simulink model "six_plus_six_AcmsteeringV09_main_2lflm"  (R2014a)
settings: Solver=FixedStepDiscrete  StartTime=0.0  StopTime=10.0  FixedStep=0.0005  RelTol=1e-3
InitFcn:
  | Veh_Par_wxt
undefined symbols (not defined in the file or in its folder): acc_spdctl, ag_thr, B, bra_em, bra_pre_gz2, bra_pre_gz34, bra_pre_yd, brakepre_dem_data, brakeTrq_dem_data, bratrq_max, ecucoder_acal, eff_tran, ESP_switch, G, guzhang_lf, guzhang_lm, guzhang_lr, guzhang_rf, guzhang_rm, guzhang_rr, kd1, kd2, ki1, ki2, kp1, kp2, L, myFIS, premax, Radius, RC_switch, s_opt_yi, s_opt_zhuan, s_opt_zhuan_add, s_opt_zhuan_table, spd_map_mot, spd_spdctl, speed_thr_park, TCS_switch, tras_ratio, trq_map_mot, trqmax_yd, trqmax_zx, trqmaxneg, v_gain, v_table, v_thr_park, zhidong_bianmazhi, zhidong_down, zhidong_up, zhidong_youmen, zhuanxiang_bianmazhi, zhuanxiang_down, zhuanxiang_up, zhuanxiang_youmen
libraries: simulink x980, ec5744lib x59, fuzblock x2
(part 21 of 25)

== system six_plus_six_AcmsteeringV09_main_2lflm/MainControl/mode_control/backward/backward/Drive/目标直驶力矩确定模块 ==
  acc_dem : Inport
  TrqLimU_dig_lf : Inport  Port=2
  TrqLimU_dig_lm : Inport  Port=3
  TrqLimU_dig_lr : Inport  Port=4
  TrqLimU_dig_rf : Inport  Port=5
  TrqLimU_dig_rm : Inport  Port=6
  TrqLimU_dig_rr : Inport  Port=7
  speed_act_lf : Inport  Port=8
  speed_act_lm : Inport  Port=9
  speed_act_lr : Inport  Port=10
  speed_act_rf : Inport  Port=11
  speed_act_rm : Inport  Port=12
  speed_act_rr : Inport  Port=13
  Add : Sum  Inputs=++++++
  Constant : Constant  Value=3.6  OutDataTypeStr=single  SampleTime=-1
  Constant1 : Constant  Value=Radius  OutDataTypeStr=single  SampleTime=-1
  Constant2 : Constant  Value=30/pi  OutDataTypeStr=single  SampleTime=-1
  Divide : Product  Inputs=*//*
  Gain : Gain  Gain=1/100
  Gain1 : Gain  Gain=tras_ratio
  Ground : Ground
  MinMax{,1..5} (6 alike) : MinMax  Inputs=2
  Product : Product
  Terminator : Terminator
  mot_map{,1..5} (6 alike) : Lookup_n-D  NumberOfTableDimensions=1  BreakpointsForDimension1=spd_map_mot  Table=trq_map_mot  InternalRulePriority=Speed  RndMeth=Simplest  InputSameDT=on
  Trq_line_dem : Outport
  wires:
  Constant1/1 -> Divide/3
  Constant/1 -> Divide/2
  Constant2/1 -> Divide/4
  Divide/1 -> Gain1/1
  TrqLimU_dig_lf/1 -> MinMax/2
  mot_map/1 -> MinMax/1
  TrqLimU_dig_lm/1 -> MinMax1/2
  TrqLimU_dig_rm/1 -> MinMax2/2
  TrqLimU_dig_rr/1 -> MinMax3/2
  Add/1 -> Product/2
  acc_dem/1 -> Gain/1
  Gain/1 -> Product/1
  Ground/1 -> Divide/1
  Gain1/1 -> Terminator/1
  speed_act_lf/1 -> mot_map/1
  speed_act_lm/1 -> mot_map1/1
  speed_act_rm/1 -> mot_map2/1
  speed_act_rr/1 -> mot_map3/1
  mot_map1/1 -> MinMax1/1
  mot_map2/1 -> MinMax2/1
  mot_map3/1 -> MinMax3/1
  Product/1 -> Trq_line_dem/1
  TrqLimU_dig_lr/1 -> MinMax4/2
  mot_map4/1 -> MinMax4/1
  TrqLimU_dig_rf/1 -> MinMax5/2
  speed_act_lr/1 -> mot_map4/1
  speed_act_rf/1 -> mot_map5/1
  mot_map5/1 -> MinMax5/1
  MinMax1/1 -> Add/2
  MinMax/1 -> Add/1
  MinMax4/1 -> Add/3
  MinMax5/1 -> Add/4
  MinMax2/1 -> Add/5
  MinMax3/1 -> Add/6

== system six_plus_six_AcmsteeringV09_main_2lflm/MainControl/mode_control/backward/backward/Drive/目标转向力矩确定模块 ==
  note: 左转为正，右转为负
  TrqLimU_dig_lf : Inport
  TrqLimU_dig_lm : Inport  Port=2
  TrqLimU_dig_lr : Inport  Port=3
  TrqLimU_dig_rf : Inport  Port=4
  TrqLimU_dig_rm : Inport  Port=5
  TrqLimU_dig_rr : Inport  Port=6
  steer_dem : Inport  Port=7
  umax : Inport  Port=8
  f : Inport  Port=9
  speed_act_lf : Inport  Port=10
  speed_act_lm : Inport  Port=11
  speed_act_lr : Inport  Port=12
  speed_act_rf : Inport  Port=13
  speed_act_rm : Inport  Port=14
  speed_act_rr : Inport  Port=15
  Add : Sum  Inputs=+++
  Add1 : Sum  Inputs=+++
  Add2 : Sum  Inputs=++++++
  Constant : Constant  Value=3.6  OutDataTypeStr=single  SampleTime=-1
  Constant1 : Constant  Value=Radius  OutDataTypeStr=single  SampleTime=-1
  Constant2 : Constant  Value=30/pi  OutDataTypeStr=single  SampleTime=-1
  Constant3 : Constant  Value=G  OutDataTypeStr=single  SampleTime=-1
  Constant4 : Constant  Value=L  OutDataTypeStr=single  SampleTime=-1
  Constant5 : Constant  Value=B  OutDataTypeStr=single  SampleTime=-1
  Constant6 : Constant  Value=eff_tran  OutDataTypeStr=single  SampleTime=-1
  Constant7 : Constant  Value=Radius  OutDataTypeStr=single  SampleTime=-1
  Constant8 : Constant  Value=ag_thr  OutDataTypeStr=single  SampleTime=-1
  Constant9 : Constant  Value=Radius  OutDataTypeStr=single  SampleTime=-1
  Divide : Product  Inputs=*//*
  Gain : Gain  Gain=1/100
  Gain1 : Gain  Gain=tras_ratio
  Gain10 : Gain  Gain=3.6
  Gain2 : Gain  Gain=tras_ratio  OutDataTypeStr=single
  Gain3 : Gain  Gain=1/tras_ratio
  Gain4 : Gain  Gain=tras_ratio  OutDataTypeStr=single
  Gain6 : Gain  Gain=1/6
  Gain7 : Gain  Gain=1/tras_ratio
  Gain8 : Gain  Gain=pi/30
  Gain9 : Gain  Gain=Radius
  Ground : Ground
  MATLAB Function : MATLAB Function  TreatAsAtomicUnit=on
  MATLAB Function1 : MATLAB Function  TreatAsAtomicUnit=on
  MATLAB Function2 : MATLAB Function  TreatAsAtomicUnit=on
  MinMax{,1..3,5..6} (6 alike) : MinMax  Inputs=2
  MinMax4 : MinMax  Function=max  Inputs=2
  Product : Product
  Terminator : Terminator
  mot_map{,1..5} (6 alike) : Lookup_n-D  NumberOfTableDimensions=1  BreakpointsForDimension1=spd_map_mot  Table=trq_map_mot  InternalRulePriority=Speed  RndMeth=Simplest  InputSameDT=on
  delta_Tsteer_dem : Outport
  wires:
  Gain/1 -> Product/1
  Product/1 -> Gain3/1
  [steer_dem] -> Gain/1
  MinMax3/1 -> Add1/2
  MinMax/1 -> Add/1
  MinMax2/1 -> Add1/1
  MinMax1/1 -> Add/2
  TrqLimU_dig_rm/1 -> MinMax3/2
  TrqLimU_dig_rf/1 -> MinMax2/2
  TrqLimU_dig_lm/1 -> MinMax1/2
  mot_map/1 -> MinMax/1
  TrqLimU_dig_lf/1 -> MinMax/2
  Divide/1 -> Gain1/1
  Constant2/1 -> Divide/4
  Constant/1 -> Divide/2
  Constant1/1 -> Divide/3
  steer_dem/1 -> [steer_dem], MATLAB Function/1(steer_dem)
  Constant3/1 -> [G], MATLAB Function/2(G)
  Constant4/1 -> [L], MATLAB Function/3(L)
  Constant5/1 -> [B], MATLAB Function/5(B)
  umax/1 -> [umax], MATLAB Function/4(umax)
  Add/1 -> Gain2/1
  Add1/1 -> Gain4/1
  Constant6/1 -> MATLAB Function/8(eff_tran)
  Constant7/1 -> MATLAB Function/9(Radius)
  f/1 -> MATLAB Function/10(f)
  MATLAB Function/1(Rturn_min) -> MinMax4/1
  [v_act] -> MATLAB Function1/1(v_act)
  Constant8/1 -> MATLAB Function1/2(ag_thr)
  MATLAB Function1/1(Rturn_min_ag) -> MinMax4/2
  [umax] -> MATLAB Function2/1(umax)
  [G] -> MATLAB Function2/2(G)
  [L] -> MATLAB Function2/3(L)
  [B] -> MATLAB Function2/4(B)
  Constant9/1 -> MATLAB Function2/5(Radius)
  MinMax4/1 -> MATLAB Function2/6(Rturn_min_xy)
  MATLAB Function2/1(delta_Tsteer_max) -> Product/2
  Ground/1 -> Divide/1
  Gain2/1 -> MATLAB Function/6(Tpeak_L)
  Gain4/1 -> MATLAB Function/7(Tpeak_R)
  speed_act_lm/1 -> Add2/2, mot_map2/1
  speed_act_rf/1 -> Add2/4, mot_map3/1
  speed_act_rm/1 -> Add2/5, mot_map4/1
  Gain1/1 -> Terminator/1
  speed_act_lf/1 -> Add2/1, mot_map/1
  mot_map2/1 -> MinMax1/1
  mot_map3/1 -> MinMax2/1
  mot_map4/1 -> MinMax3/1
  Gain3/1 -> delta_Tsteer_dem/1
  MinMax5/1 -> Add/3
  TrqLimU_dig_lr/1 -> MinMax5/2
  speed_act_lr/1 -> Add2/3, mot_map1/1
  mot_map1/1 -> MinMax5/1
  MinMax6/1 -> Add1/3
  TrqLimU_dig_rr/1 -> MinMax6/2
  speed_act_rr/1 -> Add2/6, mot_map5/1
  mot_map5/1 -> MinMax6/1
  Add2/1 -> Gain6/1
  Gain6/1 -> Gain7/1
  Gain7/1 -> Gain8/1
  Gain8/1 -> Gain9/1
  Gain9/1 -> Gain10/1
  Gain10/1 -> [v_act]

== system six_plus_six_AcmsteeringV09_main_2lflm/MainControl/mode_control/backward/backward/Drive/路面状况识别模块 ==
  In1 : Inport
  miu : Inport  Port=2
  slip_ratio : Inport  Port=3
  Signals : Inport  Port=4
  1-D Lookup Table : Lookup_n-D  NumberOfTableDimensions=1  BreakpointsForDimension1=v_table  Table=s_opt_zhuan_table  InternalRulePriority=Speed  RndMeth=Simplest  InputSameDT=on
  Abs{11..14,19..20} (6 alike) : Abs  OutDataTypeStr=single
  Bus Selector8 : BusSelector  OutputSignals=MOTOR.MOTOR1.MCU0.MCU0_SpeedFdk,MOTOR.MOTOR3.MCU0_2.MCU0_2SpeedFdk,MOTOR.MOTOR5.MCU0_4.MCU0_4SpeedFdk,MOTOR.MOTOR2.MCU0_1.MCU0_1SpeedFdk,MOTOR.MOTOR4.MCU0_3.MCU0_3SpeedFdk,MOTOR.MOTOR6.MCU0_5.MCU0_5SpeedFdk
  Constant : Constant  Value=0.9  OutDataTypeStr=single  SampleTime=-1
  Constant1 : Constant  Value=0.05  OutDataTypeStr=single  SampleTime=-1
  Constant2 : Constant  Value=s_opt_zhuan  OutDataTypeStr=single  SampleTime=-1
  Constant3 : Constant  Value=s_opt_yi  OutDataTypeStr=single  SampleTime=-1
  Gain1 : Gain  Gain=1/tras_ratio
  Gain2 : Gain  Gain=pi/30
  Gain3 : Gain  Gain=Radius
  Gain4 : Gain  Gain=3.6
  Gain5 : Gain  Gain=v_gain
  MinMax : MinMax  Inputs=6
  Terminator{,1..3} (4 alike) : Terminator
  路面识别模块 : Subsystem  Commented=on
  umax : Outport
  f : Outport  Port=2
  s_opt_zhuan : Outport  Port=3
  s_opt_yi : Outport  Port=4
  wires:
  Constant/1 -> umax/1
  Constant1/1 -> f/1
  Constant2/1 -> Terminator3/1
  Constant3/1 -> s_opt_yi/1
  In1/1 -> Terminator/1
  miu/1 -> 路面识别模块/1(miu)
  slip_ratio/1 -> 路面识别模块/2(slip_ratio)
  路面识别模块/1(best_slip_ratio) -> Terminator1/1
  路面识别模块/2(max_miu) -> Terminator2/1
  Signals/1 -> Bus Selector8/1
  Abs12/1 -> MinMax/2
  Abs11/1 -> MinMax/1
  Abs13/1 -> MinMax/3
  Abs14/1 -> MinMax/4
  Abs19/1 -> MinMax/5
  Abs20/1 -> MinMax/6
  Bus Selector8/2 -> Abs12/1  "<MCU0_2SpeedFdk>"
  Bus Selector8/1 -> Abs11/1  "<MCU0_SpeedFdk>"
  Bus Selector8/3 -> Abs13/1  "<MCU0_4SpeedFdk>"
  Bus Selector8/4 -> Abs14/1  "<MCU0_1SpeedFdk>"
  Bus Selector8/5 -> Abs19/1  "<MCU0_3SpeedFdk>"
  Bus Selector8/6 -> Abs20/1  "<MCU0_5SpeedFdk>"
  MinMax/1 -> Gain1/1
  Gain1/1 -> Gain2/1
  Gain2/1 -> Gain3/1
  Gain3/1 -> Gain4/1
  Gain4/1 -> Gain5/1
  Gain5/1 -> 1-D Lookup Table/1
  1-D Lookup Table/1 -> s_opt_zhuan/1

== system six_plus_six_AcmsteeringV09_main_2lflm/MainControl/mode_control/backward/backward/Drive/车辆稳定性控制 ==
  note: 加速度向左为正
  acc_y : Inport
  Action Port : ActionPort  ActionType=case
  Abs : Abs
  Add10 : Sum  Inputs=+-+
  Add2 : Sum  Inputs=+++
  Constant : Constant  Value=ag_thr  OutDataTypeStr=single  SampleTime=-1
  Constant1 : Constant  OutDataTypeStr=int8  SampleTime=-1
  Constant2 : Constant  Value=-1  OutDataTypeStr=int8  SampleTime=-1
  Constant3 : Constant  Value=ESP_switch  OutDataTypeStr=single  SampleTime=-1
  Constant4 : Constant  Value=0  OutDataTypeStr=single  SampleTime=-1
  Gain20 : Gain  Gain=2
  Gain3 : Gain  Gain=1/tras_ratio
  Gain5 : Gain  Gain=kp1  OutDataTypeStr=single
  Gain6 : Gain  Gain=ki1  OutDataTypeStr=single
  Gain7 : Gain  Gain=kd1  OutDataTypeStr=single
  Memory{3..5,13} (4 alike) : Memory  InheritSampleTime=on
  Product : Product  OutDataTypeStr=single
  Subtract1 : Sum  Inputs=+-
  Subtract5 : Sum
  Sum : Sum  Inputs=|+-
  Switch : Switch
  Switch1 : Switch  Criteria=u2 > Threshold  Threshold=0.5
  delta_Twending_dem : Outport
  wires:
  Constant/1 -> Sum/1
  acc_y/1 -> Switch/2, Abs/1
  Abs/1 -> Sum/2
  Constant1/1 -> Switch/1
  Constant2/1 -> Switch/3
  Switch/1 -> Product/2
  Product/1 -> Gain3/1
  Constant3/1 -> Switch1/2
  Switch1/1 -> delta_Twending_dem/1
  Constant4/1 -> Switch1/3
  Sum/1 -> Memory4/1, Add10/1, Gain6/1, Memory3/1, Subtract1/1
  Gain5/1 -> Add2/1
  Gain6/1 -> Add2/2
  Memory3/1 -> Subtract1/2
  Add10/1 -> Gain7/1
  Gain20/1 -> Add10/2
  Memory5/1 -> Add10/3
  Gain7/1 -> Add2/3
  Subtract1/1 -> Gain5/1
  Memory4/1 -> Memory5/1, Gain20/1
  Add2/1 -> Subtract5/1
  Subtract5/1 -> Product/1, Memory13/1
  Memory13/1 -> Subtract5/2
  Gain3/1 -> Switch1/1

== system six_plus_six_AcmsteeringV09_main_2lflm/MainControl/mode_control/backward/backward/Drive/车辆稳定性控制1 ==
  Action Port : ActionPort  ActionType=case
  Constant4 : Constant  Value=0  OutDataTypeStr=single  SampleTime=-1
  1 : Outport
  wires:
  Constant4/1 -> 1/1

== system six_plus_six_AcmsteeringV09_main_2lflm/MainControl/mode_control/backward/backward/Drive/驱动防滑控制TCS ==
  trq_dem_lf : Inport
  trq_dem_lm : Inport  Port=2
  trq_dem_lr : Inport  Port=3
  trq_dem_rf : Inport  Port=4
  trq_dem_rm : Inport  Port=5
  trq_dem_rr : Inport  Port=6
  bra_pre_l : Inport  Port=7
  bra_pre_r : Inport  Port=8
  speed_act_lf : Inport  Port=9
  speed_act_lm : Inport  Port=10
  speed_act_lr : Inport  Port=11
  speed_act_rf : Inport  Port=12
  speed_act_rm : Inport  Port=13
  speed_act_rr : Inport  Port=14
  v_act : Inport  Port=15
  brake_dem : Inport  Port=16
  s_opt_zhuan : Inport  Port=17
  Signals : Inport  Port=18
  直行TCS : Subsystem  TreatAsAtomicUnit=on
  backward_dem : Outport
  wires:
  直行TCS/1(backward_dem) -> backward_dem/1
  trq_dem_lf/1 -> 直行TCS/1(trq_dem_lf)
  trq_dem_lm/1 -> 直行TCS/2(trq_dem_lm)
  trq_dem_lr/1 -> 直行TCS/3(trq_dem_lr)
  trq_dem_rf/1 -> 直行TCS/4(trq_dem_rf)
  trq_dem_rm/1 -> 直行TCS/5(trq_dem_rm)
  trq_dem_rr/1 -> 直行TCS/6(trq_dem_rr)
  bra_pre_l/1 -> 直行TCS/7(bra_pre_l)
  bra_pre_r/1 -> 直行TCS/8(bra_pre_r)
  brake_dem/1 -> 直行TCS/16(brake_dem)
  Signals/1 -> 直行TCS/18(Signals)
  speed_act_rr/1 -> 直行TCS/14(speed_act_rr)
  speed_act_rm/1 -> 直行TCS/13(speed_act_rm)
  v_act/1 -> 直行TCS/15(v_act)
  speed_act_rf/1 -> 直行TCS/12(speed_act_rf)
  speed_act_lr/1 -> 直行TCS/11(speed_act_lr)
  speed_act_lm/1 -> 直行TCS/10(speed_act_lm)
  speed_act_lf/1 -> 直行TCS/9(speed_act_lf)
  s_opt_zhuan/1 -> 直行TCS/17(s_opt_zhuan)

== system six_plus_six_AcmsteeringV09_main_2lflm/MainControl/mode_control/forward/forward/Brake/Subsystem ==
  MCU2 : Inport
  Bus Selector : BusSelector  OutputSignals=MCU2_MotorStallingFault,MCU2_UdcDetectionFault,MCU2_TempSensorFault,MCU2_ActiveDischargingFault,MCU2_ldcSensorFault,MCU2_luSensorFault,MCU2_lvSensorFault,MCU2_FaultLevel,MCU2_Controllerload,MCU2_CanCommunicationFault,MCU2_MemoryFault,MCU2_DownratingFault,MCU2_IGBTFault,MCU2_MotorOverTemp,MCU2_ControllerOverTemp,MCU2_MotorOverSpeed,MCU2_RotaryInverterFault,MCU2_UnderVoltage,MCU2_OverVoltage,MCU2_MotorOverLoad
  Compare To Constant{,1..19} (20 alike) : simulink/Logic and Bit Operations/Compare To Constant  relop===  const=1  OutDataTypeStr=boolean
  Logical Operator : Logic  Operator=OR  Inputs=20  AllPortsSameDT=off  OutDataTypeStr=boolean
  guzhang_lf : Outport
  wires:
  MCU2/1 -> Bus Selector/1
  Bus Selector/1 -> Compare To Constant/1  "<MCU2_MotorStallingFault>"
  Bus Selector/2 -> Compare To Constant1/1  "<MCU2_UdcDetectionFault>"
  Bus Selector/3 -> Compare To Constant2/1  "<MCU2_TempSensorFault>"
  Bus Selector/4 -> Compare To Constant3/1  "<MCU2_ActiveDischargingFault>"
  Bus Selector/5 -> Compare To Constant4/1  "<MCU2_ldcSensorFault>"
  Bus Selector/6 -> Compare To Constant5/1  "<MCU2_luSensorFault>"
  Bus Selector/7 -> Compare To Constant6/1  "<MCU2_lvSensorFault>"
  Bus Selector/8 -> Compare To Constant7/1  "<MCU2_FaultLevel>"
  Bus Selector/13 -> Compare To Constant12/1  "<MCU2_IGBTFault>"
  Bus Selector/14 -> Compare To Constant13/1  "<MCU2_MotorOverTemp>"
  Bus Selector/10 -> Compare To Constant9/1  "<MCU2_CanCommunicationFault>"
  Bus Selector/16 -> Compare To Constant15/1  "<MCU2_MotorOverSpeed>"
  Bus Selector/11 -> Compare To Constant10/1  "<MCU2_MemoryFault>"
  Bus Selector/15 -> Compare To Constant14/1  "<MCU2_ControllerOverTemp>"
  Bus Selector/12 -> Compare To Constant11/1  "<MCU2_DownratingFault>"
  Bus Selector/9 -> Compare To Constant8/1  "<MCU2_Controllerload>"
  Bus Selector/18 -> Compare To Constant17/1  "<MCU2_UnderVoltage>"
  Bus Selector/20 -> Compare To Constant19/1  "<MCU2_MotorOverLoad>"
  Bus Selector/19 -> Compare To Constant18/1  "<MCU2_OverVoltage>"
  Bus Selector/17 -> Compare To Constant16/1  "<MCU2_RotaryInverterFault>"
  Compare To Constant9/1 -> Logical Operator/10
  Compare To Constant12/1 -> Logical Operator/13
  Compare To Constant11/1 -> Logical Operator/12
  Compare To Constant15/1 -> Logical Operator/16
  Compare To Constant8/1 -> Logical Operator/9
  Compare To Constant10/1 -> Logical Operator/11
  Compare To Constant13/1 -> Logical Operator/14
  Compare To Constant14/1 -> Logical Operator/15
  Compare To Constant1/1 -> Logical Operator/2
  Compare To Constant17/1 -> Logical Operator/18
  Compare To Constant16/1 -> Logical Operator/17
  Compare To Constant18/1 -> Logical Operator/19
  Compare To Constant19/1 -> Logical Operator/20
  Compare To Constant3/1 -> Logical Operator/4
  Compare To Constant2/1 -> Logical Operator/3
  Compare To Constant6/1 -> Logical Operator/7
  Compare To Constant4/1 -> Logical Operator/5
  Compare To Constant5/1 -> Logical Operator/6
  Compare To Constant7/1 -> Logical Operator/8
  Compare To Constant/1 -> Logical Operator/1
  Logical Operator/1 -> guzhang_lf/1

== system six_plus_six_AcmsteeringV09_main_2lflm/MainControl/mode_control/forward/forward/Brake/Subsystem1 ==
  speed_act_lf : Inport
  speed_act_lm : Inport  Port=2
  speed_act_lr : Inport  Port=3
  speed_act_rf : Inport  Port=4
  speed_act_rm : Inport  Port=5
  speed_act_rr : Inport  Port=6
  mot_map{,1..5} (6 alike) : Lookup_n-D  NumberOfTableDimensions=1  BreakpointsForDimension1=spd_map_mot  Table=trq_map_mot  InternalRulePriority=Speed  RndMeth=Simplest  InputSameDT=on
  trqlim_map_lf : Outport
  trqlim_map_lm : Outport  Port=2
  trqlim_map_lr : Outport  Port=3
  trqlim_map_rf : Outport  Port=4
  trqlim_map_rm : Outport  Port=5
  trqlim_map_rr : Outport  Port=6
  wires:
  speed_act_lf/1 -> mot_map/1
  speed_act_lr/1 -> mot_map1/1
  speed_act_rf/1 -> mot_map2/1
  speed_act_rr/1 -> mot_map3/1
  mot_map/1 -> trqlim_map_lf/1
  mot_map1/1 -> trqlim_map_lr/1
  mot_map2/1 -> trqlim_map_rf/1
  mot_map3/1 -> trqlim_map_rr/1
  speed_act_lm/1 -> mot_map4/1
  mot_map4/1 -> trqlim_map_lm/1
  speed_act_rm/1 -> mot_map5/1
  mot_map5/1 -> trqlim_map_rm/1

== system six_plus_six_AcmsteeringV09_main_2lflm/MainControl/mode_control/forward/forward/Brake/Subsystem2 ==
  MCU2_2 : Inport
  Bus Selector : BusSelector  OutputSignals=MCU2_2MotorStallingFault,MCU2_2UdcDetectionFault,MCU2_2TempSensorFault,MCU2_2ActiveDischargingFault,MCU2_2ldcSensorFault,MCU2_2luSensorFault,MCU2_2lvSensorFault,MCU2_2FaultLevel,MCU2_2Controllerload,MCU2_2CanCommunicationFault,MCU2_2MemoryFault,MCU2_2DownratingFault,MCU2_2IGBTFault,MCU2_2MotorOverTemp,MCU2_2ControllerOverTemp,MCU2_2MotorOverSpeed,MCU2_2RotaryInverterFault,MCU2_2UnderVoltage,MCU2_OverVoltage,MCU2_2MotorOverLoad
  Compare To Constant{,1..19} (20 alike) : simulink/Logic and Bit Operations/Compare To Constant  relop===  const=1  OutDataTypeStr=boolean
  Logical Operator : Logic  Operator=OR  Inputs=20  AllPortsSameDT=off  OutDataTypeStr=boolean
  guzhang_lm : Outport
  wires:
  Logical Operator/1 -> guzhang_lm/1
  Compare To Constant/1 -> Logical Operator/1
  Compare To Constant7/1 -> Logical Operator/8
  Compare To Constant5/1 -> Logical Operator/6
  Compare To Constant4/1 -> Logical Operator/5
  Compare To Constant6/1 -> Logical Operator/7
  Compare To Constant2/1 -> Logical Operator/3
  Compare To Constant3/1 -> Logical Operator/4
  Compare To Constant19/1 -> Logical Operator/20
  Compare To Constant18/1 -> Logical Operator/19
  Compare To Constant16/1 -> Logical Operator/17
  Compare To Constant17/1 -> Logical Operator/18
  Compare To Constant1/1 -> Logical Operator/2
  Compare To Constant14/1 -> Logical Operator/15
  Compare To Constant13/1 -> Logical Operator/14
  Compare To Constant10/1 -> Logical Operator/11
  Compare To Constant8/1 -> Logical Operator/9
  Compare To Constant15/1 -> Logical Operator/16
  Compare To Constant11/1 -> Logical Operator/12
  Compare To Constant12/1 -> Logical Operator/13
  Compare To Constant9/1 -> Logical Operator/10
  Bus Selector/17 -> Compare To Constant16/1  "<MCU2_2RotaryInverterFault>"
  Bus Selector/19 -> Compare To Constant18/1  "<MCU2_OverVoltage>"
  Bus Selector/20 -> Compare To Constant19/1  "<MCU2_2MotorOverLoad>"
  Bus Selector/18 -> Compare To Constant17/1  "<MCU2_2UnderVoltage>"
  Bus Selector/9 -> Compare To Constant8/1  "<MCU2_2Controllerload>"
  Bus Selector/12 -> Compare To Constant11/1  "<MCU2_2DownratingFault>"
  Bus Selector/15 -> Compare To Constant14/1  "<MCU2_2ControllerOverTemp>"
  Bus Selector/11 -> Compare To Constant10/1  "<MCU2_2MemoryFault>"
  Bus Selector/16 -> Compare To Constant15/1  "<MCU2_2MotorOverSpeed>"
  Bus Selector/10 -> Compare To Constant9/1  "<MCU2_2CanCommunicationFault>"
  Bus Selector/14 -> Compare To Constant13/1  "<MCU2_2MotorOverTemp>"
  Bus Selector/13 -> Compare To Constant12/1  "<MCU2_2IGBTFault>"
  Bus Selector/8 -> Compare To Constant7/1  "<MCU2_2FaultLevel>"
  Bus Selector/7 -> Compare To Constant6/1  "<MCU2_2lvSensorFault>"
  Bus Selector/6 -> Compare To Constant5/1  "<MCU2_2luSensorFault>"
  Bus Selector/5 -> Compare To Constant4/1  "<MCU2_2ldcSensorFault>"
  Bus Selector/4 -> Compare To Constant3/1  "<MCU2_2ActiveDischargingFault>"
  Bus Selector/3 -> Compare To Constant2/1  "<MCU2_2TempSensorFault>"
  Bus Selector/2 -> Compare To Constant1/1  "<MCU2_2UdcDetectionFault>"
  Bus Selector/1 -> Compare To Constant/1  "<MCU2_2MotorStallingFault>"
  MCU2_2/1 -> Bus Selector/1

== matlab function six_plus_six_AcmsteeringV09_main_2lflm/MainControl/mode_control/emergency_stop/emergency_stop/HeartBeat ==
  data: life_pre input; life output
function life = fcn(life_pre)
%#codegen
life=single(life_pre+1);
if life>255
    life=single(0);
end
end

== matlab function six_plus_six_AcmsteeringV09_main_2lflm/MainControl/mode_control/emergency_stop/emergency_stop/HeartBeat4 ==
  data: life_pre input; life output
function life = fcn(life_pre)
%#codegen
life=single(life_pre+1);
if life>255
    life=single(0);
end
end

== matlab function six_plus_six_AcmsteeringV09_main_2lflm/Data_input/2/Enabled Subsystem/MATLAB Function1 ==
  data: current_in input; current_out output
function current_out = motec_current(current_in)
    if current_in>32768
        current_out=current_in-65535;
    else
        current_out=current_in;
    end
end

== matlab function six_plus_six_AcmsteeringV09_main_2lflm/MainControl/mode_control/forward/forward/Drive/驱动防滑控制TCS/直行TCS/直行/MATLAB Function2 ==
  data: s_act_rf input; flag_rf output; s_opt_zhuan input; s_opt_zhuan_add input; flag_rf_pre input int8
function flag_rf = fcn(s_act_rf,s_opt_zhuan,s_opt_zhuan_add,flag_rf_pre)
%#codegen
if s_act_rf>s_opt_zhuan+s_opt_zhuan_add
    flag_rf=int8(1);
elseif s_act_rf<s_opt_zhuan
    flag_rf =int8(0);
else
    flag_rf=int8(flag_rf_pre);
end
end

== matlab function six_plus_six_AcmsteeringV09_main_2lflm/MainControl/mode_control/backward/backward/Drive/驱动防滑控制TCS/直行TCS/直行/MATLAB Function1 ==
  data: s_act_lr input; flag_lr output; s_opt_zhuan input; s_opt_zhuan_add input; flag_lr_pre input int8
function flag_lr = fcn(s_act_lr,s_opt_zhuan,s_opt_zhuan_add,flag_lr_pre)
%#codegen
if s_act_lr>s_opt_zhuan+s_opt_zhuan_add
    flag_lr=int8(1);
elseif s_act_lr<s_opt_zhuan
    flag_lr =int8(0);
else
    flag_lr=int8(flag_lr_pre);
end
end

== matlab function six_plus_six_AcmsteeringV09_main_2lflm/Subsystem/MATLAB Function ==
  data: data_1 input; data output; data_2 input; zero output; position_4 output; position_3 output; position_2 output; position_1 output
function [data,zero,position_4,position_3,position_2,position_1] = motec_write(data_1,data_2)
if  data_1<150
    if (mod(data_1,6)<3)
    data=6;
    else
    data=7;
    end
    zero=hex2dec('00');
    position_1=hex2dec('00');
    position_2=hex2dec('00');
    position_3=hex2dec('00');
    position_4=hex2dec('00');  
else
    if (mod(data_1,2)==0)
        data=15;
        zero=hex2dec('00');
    else
        zero=hex2dec('00');
        data=95;    
    end
%Negative numbers are represented with the Two's Complement
       data_2=double(data_2);
       if data_2<0
       data_2= 2^32+data_2;
       end
%Find the 4 bytes
       position_1= floor( data_2/(2^24) );
       remainder1     = floor( mod( data_2,(2^24) ) );
       position_2= floor( remainder1/(2^16) );
       remainder2     = floor( mod( remainder1,(2^16) ) );
       position_3= floor( remainder2/(2^8) );
       position_4= floor( mod( remainder2,(2^8) ) );
 
end

== system six_plus_six_AcmsteeringV09_main_2lflm/MainControl/mode_control/forward/forward/Brake/Subsystem3 ==
  MCU2_4 : Inport
  Bus Selector : BusSelector  OutputSignals=MCU2_4MotorStallingFault,MCU2_4UdcDetectionFault,MCU2_4TempSensorFault,MCU2_4ActiveDischargingFault,MCU2_4ldcSensorFault,MCU2_4luSensorFault,MCU2_4lvSensorFault,MCU2_4FaultLevel,MCU2_4Controllerload,MCU2_4CanCommunicationFault,MCU2_4MemoryFault,MCU2_4DownratingFault,MCU2_4IGBTFault,MCU2_4MotorOverTemp,MCU2_4ControllerOverTemp,MCU2_4MotorOverSpeed,MCU2_4RotaryInverterFault,MCU2_4UnderVoltage,MCU2_4OverVoltage,MCU2_4MotorOverLoad
  Compare To Constant{,1..19} (20 alike) : simulink/Logic and Bit Operations/Compare To Constant  relop===  const=1  OutDataTypeStr=boolean
  Logical Operator : Logic  Operator=OR  Inputs=20  AllPortsSameDT=off  OutDataTypeStr=boolean
  guzhang_lr : Outport
  wires:
  MCU2_4/1 -> Bus Selector/1
  Bus Selector/1 -> Compare To Constant/1  "<MCU2_4MotorStallingFault>"
  Bus Selector/2 -> Compare To Constant1/1  "<MCU2_4UdcDetectionFault>"
  Bus Selector/3 -> Compare To Constant2/1  "<MCU2_4TempSensorFault>"
  Bus Selector/4 -> Compare To Constant3/1  "<MCU2_4ActiveDischargingFault>"
  Bus Selector/5 -> Compare To Constant4/1  "<MCU2_4ldcSensorFault>"
  Bus Selector/6 -> Compare To Constant5/1  "<MCU2_4luSensorFault>"
  Bus Selector/7 -> Compare To Constant6/1  "<MCU2_4lvSensorFault>"
  Bus Selector/8 -> Compare To Constant7/1  "<MCU2_4FaultLevel>"
  Bus Selector/13 -> Compare To Constant12/1  "<MCU2_4IGBTFault>"
  Bus Selector/14 -> Compare To Constant13/1  "<MCU2_4MotorOverTemp>"
  Bus Selector/10 -> Compare To Constant9/1  "<MCU2_4CanCommunicationFault>"
  Bus Selector/16 -> Compare To Constant15/1  "<MCU2_4MotorOverSpeed>"
  Bus Selector/11 -> Compare To Constant10/1  "<MCU2_4MemoryFault>"
  Bus Selector/15 -> Compare To Constant14/1  "<MCU2_4ControllerOverTemp>"
  Bus Selector/12 -> Compare To Constant11/1  "<MCU2_4DownratingFault>"
  Bus Selector/9 -> Compare To Constant8/1  "<MCU2_4Controllerload>"
  Bus Selector/18 -> Compare To Constant17/1  "<MCU2_4UnderVoltage>"
  Bus Selector/20 -> Compare To Constant19/1  "<MCU2_4MotorOverLoad>"
  Bus Selector/19 -> Compare To Constant18/1  "<MCU2_4OverVoltage>"
  Bus Selector/17 -> Compare To Constant16/1  "<MCU2_4RotaryInverterFault>"
  Compare To Constant9/1 -> Logical Operator/10
  Compare To Constant12/1 -> Logical Operator/13
  Compare To Constant11/1 -> Logical Operator/12
  Compare To Constant15/1 -> Logical Operator/16
  Compare To Constant8/1 -> Logical Operator/9
  Compare To Constant10/1 -> Logical Operator/11
  Compare To Constant13/1 -> Logical Operator/14
  Compare To Constant14/1 -> Logical Operator/15
  Compare To Constant1/1 -> Logical Operator/2
  Compare To Constant17/1 -> Logical Operator/18
  Compare To Constant16/1 -> Logical Operator/17
  Compare To Constant18/1 -> Logical Operator/19
  Compare To Constant19/1 -> Logical Operator/20
  Compare To Constant3/1 -> Logical Operator/4
  Compare To Constant2/1 -> Logical Operator/3
  Compare To Constant6/1 -> Logical Operator/7
  Compare To Constant4/1 -> Logical Operator/5
  Compare To Constant5/1 -> Logical Operator/6
  Compare To Constant7/1 -> Logical Operator/8
  Compare To Constant/1 -> Logical Operator/1
  Logical Operator/1 -> guzhang_lr/1

== system six_plus_six_AcmsteeringV09_main_2lflm/MainControl/mode_control/forward/forward/Brake/Subsystem4 ==
  MCU2_1 : Inport
  Bus Selector : BusSelector  OutputSignals=MCU2_1MotorStallingFault,MCU2_1UdcDetectionFault,MCU2_1TempSensorFault,MCU2_1ActiveDischargingFault,MCU2_1ldcSensorFault,MCU2_1luSensorFault,MCU2_1lvSensorFault,MCU2_1FaultLevel,MCU2_1Controllerload,MCU2_1CanCommunicationFault,MCU2_1MemoryFault,MCU2_1DownratingFault,MCU2_1IGBTFault,MCU2_1MotorOverTemp,MCU2_1ControllerOverTemp,MCU2_1MotorOverSpeed,MCU2_1RotaryInverterFault,MCU2_1UnderVoltage,MCU2_1OverVoltage,MCU2_1MotorOverLoad
  Compare To Constant{,1..19} (20 alike) : simulink/Logic and Bit Operations/Compare To Constant  relop===  const=1  OutDataTypeStr=boolean
  Logical Operator : Logic  Operator=OR  Inputs=20  AllPortsSameDT=off  OutDataTypeStr=boolean
  guzhang_rf : Outport
  wires:
  Logical Operator/1 -> guzhang_rf/1
  Compare To Constant/1 -> Logical Operator/1
  Compare To Constant7/1 -> Logical Operator/8
  Compare To Constant5/1 -> Logical Operator/6
  Compare To Constant4/1 -> Logical Operator/5
  Compare To Constant6/1 -> Logical Operator/7
  Compare To Constant2/1 -> Logical Operator/3
  Compare To Constant3/1 -> Logical Operator/4
  Compare To Constant19/1 -> Logical Operator/20
  Compare To Constant18/1 -> Logical Operator/19
  Compare To Constant16/1 -> Logical Operator/17
  Compare To Constant17/1 -> Logical Operator/18
  Compare To Constant1/1 -> Logical Operator/2
  Compare To Constant14/1 -> Logical Operator/15
  Compare To Constant13/1 -> Logical Operator/14
  Compare To Constant10/1 -> Logical Operator/11
  Compare To Constant8/1 -> Logical Operator/9
  Compare To Constant15/1 -> Logical Operator/16
  Compare To Constant11/1 -> Logical Operator/12
  Compare To Constant12/1 -> Logical Operator/13
  Compare To Constant9/1 -> Logical Operator/10
  Bus Selector/17 -> Compare To Constant16/1  "<MCU2_1RotaryInverterFault>"
  Bus Selector/19 -> Compare To Constant18/1  "<MCU2_1OverVoltage>"
  Bus Selector/20 -> Compare To Constant19/1  "<MCU2_1MotorOverLoad>"
  Bus Selector/18 -> Compare To Constant17/1  "<MCU2_1UnderVoltage>"
  Bus Selector/9 -> Compare To Constant8/1  "<MCU2_1Controllerload>"
  Bus Selector/12 -> Compare To Constant11/1  "<MCU2_1DownratingFault>"
  Bus Selector/15 -> Compare To Constant14/1  "<MCU2_1ControllerOverTemp>"
  Bus Selector/11 -> Compare To Constant10/1  "<MCU2_1MemoryFault>"
  Bus Selector/16 -> Compare To Constant15/1  "<MCU2_1MotorOverSpeed>"
  Bus Selector/10 -> Compare To Constant9/1  "<MCU2_1CanCommunicationFault>"
  Bus Selector/14 -> Compare To Constant13/1  "<MCU2_1MotorOverTemp>"
  Bus Selector/13 -> Compare To Constant12/1  "<MCU2_1IGBTFault>"
  Bus Selector/8 -> Compare To Constant7/1  "<MCU2_1FaultLevel>"
  Bus Selector/7 -> Compare To Constant6/1  "<MCU2_1lvSensorFault>"
  Bus Selector/6 -> Compare To Constant5/1  "<MCU2_1luSensorFault>"
  Bus Selector/5 -> Compare To Constant4/1  "<MCU2_1ldcSensorFault>"
  Bus Selector/4 -> Compare To Constant3/1  "<MCU2_1ActiveDischargingFault>"
  Bus Selector/3 -> Compare To Constant2/1  "<MCU2_1TempSensorFault>"
  Bus Selector/2 -> Compare To Constant1/1  "<MCU2_1UdcDetectionFault>"
  Bus Selector/1 -> Compare To Constant/1  "<MCU2_1MotorStallingFault>"
  MCU2_1/1 -> Bus Selector/1

== system six_plus_six_AcmsteeringV09_main_2lflm/MainControl/mode_control/forward/forward/Brake/Subsystem5 ==
  MCU2_3 : Inport
  Bus Selector : BusSelector  OutputSignals=MCU2_3MotorStallingFault,MCU2_3UdcDetectionFault,MCU2_3TempSensorFault,MCU2_3ActiveDischargingFault,MCU2_3ldcSensorFault,MCU2_3luSensorFault,MCU2_3lvSensorFault,MCU2_3FaultLevel,MCU2_3Controllerload,MCU2_3CanCommunicationFault,MCU2_3MemoryFault,MCU2_3DownratingFault,MCU2_3IGBTFault,MCU2_3MotorOverTemp,MCU2_3ControllerOverTemp,MCU2_3MotorOverSpeed,MCU2_3RotaryInverterFault,MCU2_3UnderVoltage,MCU2_3OverVoltage,MCU2_3MotorOverLoad
  Compare To Constant{,1..19} (20 alike) : simulink/Logic and Bit Operations/Compare To Constant  relop===  const=1  OutDataTypeStr=boolean
  Logical Operator : Logic  Operator=OR  Inputs=20  AllPortsSameDT=off  OutDataTypeStr=boolean
  guzhang_rm : Outport
  wires:
  MCU2_3/1 -> Bus Selector/1
  Bus Selector/1 -> Compare To Constant/1  "<MCU2_3MotorStallingFault>"
  Bus Selector/2 -> Compare To Constant1/1  "<MCU2_3UdcDetectionFault>"
  Bus Selector/3 -> Compare To Constant2/1  "<MCU2_3TempSensorFault>"
  Bus Selector/4 -> Compare To Constant3/1  "<MCU2_3ActiveDischargingFault>"
  Bus Selector/5 -> Compare To Constant4/1  "<MCU2_3ldcSensorFault>"
  Bus Selector/6 -> Compare To Constant5/1  "<MCU2_3luSensorFault>"
  Bus Selector/7 -> Compare To Constant6/1  "<MCU2_3lvSensorFault>"
  Bus Selector/8 -> Compare To Constant7/1  "<MCU2_3FaultLevel>"
  Bus Selector/13 -> Compare To Constant12/1  "<MCU2_3IGBTFault>"
  Bus Selector/14 -> Compare To Constant13/1  "<MCU2_3MotorOverTemp>"
  Bus Selector/10 -> Compare To Constant9/1  "<MCU2_3CanCommunicationFault>"
  Bus Selector/16 -> Compare To Constant15/1  "<MCU2_3MotorOverSpeed>"
  Bus Selector/11 -> Compare To Constant10/1  "<MCU2_3MemoryFault>"
  Bus Selector/15 -> Compare To Constant14/1  "<MCU2_3ControllerOverTemp>"
  Bus Selector/12 -> Compare To Constant11/1  "<MCU2_3DownratingFault>"
  Bus Selector/9 -> Compare To Constant8/1  "<MCU2_3Controllerload>"
  Bus Selector/18 -> Compare To Constant17/1  "<MCU2_3UnderVoltage>"
  Bus Selector/20 -> Compare To Constant19/1  "<MCU2_3MotorOverLoad>"
  Bus Selector/19 -> Compare To Constant18/1  "<MCU2_3OverVoltage>"
  Bus Selector/17 -> Compare To Constant16/1  "<MCU2_3RotaryInverterFault>"
  Compare To Constant9/1 -> Logical Operator/10
  Compare To Constant12/1 -> Logical Operator/13
  Compare To Constant11/1 -> Logical Operator/12
  Compare To Constant15/1 -> Logical Operator/16
  Compare To Constant8/1 -> Logical Operator/9
  Compare To Constant10/1 -> Logical Operator/11
  Compare To Constant13/1 -> Logical Operator/14
  Compare To Constant14/1 -> Logical Operator/15
  Compare To Constant1/1 -> Logical Operator/2
  Compare To Constant17/1 -> Logical Operator/18
  Compare To Constant16/1 -> Logical Operator/17
  Compare To Constant18/1 -> Logical Operator/19
  Compare To Constant19/1 -> Logical Operator/20
  Compare To Constant3/1 -> Logical Operator/4
  Compare To Constant2/1 -> Logical Operator/3
  Compare To Constant6/1 -> Logical Operator/7
  Compare To Constant4/1 -> Logical Operator/5
  Compare To Constant5/1 -> Logical Operator/6
  Compare To Constant7/1 -> Logical Operator/8
  Compare To Constant/1 -> Logical Operator/1
  Logical Operator/1 -> guzhang_rm/1

== system six_plus_six_AcmsteeringV09_main_2lflm/MainControl/mode_control/forward/forward/Brake/Subsystem6 ==
  MCU2_5 : Inport
  Bus Selector : BusSelector  OutputSignals=MCU2_5MotorStallingFault,MCU2_5UdcDetectionFault,MCU2_5TempSensorFault,MCU2_5ActiveDischargingFault,MCU2_5ldcSensorFault,MCU2_5luSensorFault,MCU2_5lvSensorFault,MCU2_5FaultLevel,MCU2_5Controllerload,MCU2_5CanCommunicationFault,MCU2_5MemoryFault,MCU2_5DownratingFault,MCU2_5IGBTFault,MCU2_5MotorOverTemp,MCU2_5ControllerOverTemp,MCU2_5MotorOverSpeed,MCU2_5RotaryInverterFault,MCU2_5UnderVoltage,MCU2_5OverVoltage,MCU2_5MotorOverLoad
  Compare To Constant{,1..19} (20 alike) : simulink/Logic and Bit Operations/Compare To Constant  relop===  const=1  OutDataTypeStr=boolean
  Logical Operator : Logic  Operator=OR  Inputs=20  AllPortsSameDT=off  OutDataTypeStr=boolean
  guzhang_rr : Outport
  wires:
  Logical Operator/1 -> guzhang_rr/1
  Compare To Constant/1 -> Logical Operator/1
  Compare To Constant7/1 -> Logical Operator/8
  Compare To Constant5/1 -> Logical Operator/6
  Compare To Constant4/1 -> Logical Operator/5
  Compare To Constant6/1 -> Logical Operator/7
  Compare To Constant2/1 -> Logical Operator/3
  Compare To Constant3/1 -> Logical Operator/4
  Compare To Constant19/1 -> Logical Operator/20
  Compare To Constant18/1 -> Logical Operator/19
  Compare To Constant16/1 -> Logical Operator/17
  Compare To Constant17/1 -> Logical Operator/18
  Compare To Constant1/1 -> Logical Operator/2
  Compare To Constant14/1 -> Logical Operator/15
  Compare To Constant13/1 -> Logical Operator/14
  Compare To Constant10/1 -> Logical Operator/11
  Compare To Constant8/1 -> Logical Operator/9
  Compare To Constant15/1 -> Logical Operator/16
  Compare To Constant11/1 -> Logical Operator/12
  Compare To Constant12/1 -> Logical Operator/13
  Compare To Constant9/1 -> Logical Operator/10
  Bus Selector/17 -> Compare To Constant16/1  "<MCU2_5RotaryInverterFault>"
  Bus Selector/19 -> Compare To Constant18/1  "<MCU2_5OverVoltage>"
  Bus Selector/20 -> Compare To Constant19/1  "<MCU2_5MotorOverLoad>"
  Bus Selector/18 -> Compare To Constant17/1  "<MCU2_5UnderVoltage>"
  Bus Selector/9 -> Compare To Constant8/1  "<MCU2_5Controllerload>"
  Bus Selector/12 -> Compare To Constant11/1  "<MCU2_5DownratingFault>"
  Bus Selector/15 -> Compare To Constant14/1  "<MCU2_5ControllerOverTemp>"
  Bus Selector/11 -> Compare To Constant10/1  "<MCU2_5MemoryFault>"
  Bus Selector/16 -> Compare To Constant15/1  "<MCU2_5MotorOverSpeed>"
  Bus Selector/10 -> Compare To Constant9/1  "<MCU2_5CanCommunicationFault>"
  Bus Selector/14 -> Compare To Constant13/1  "<MCU2_5MotorOverTemp>"
  Bus Selector/13 -> Compare To Constant12/1  "<MCU2_5IGBTFault>"
  Bus Selector/8 -> Compare To Constant7/1  "<MCU2_5FaultLevel>"
  Bus Selector/7 -> Compare To Constant6/1  "<MCU2_5lvSensorFault>"
  Bus Selector/6 -> Compare To Constant5/1  "<MCU2_5luSensorFault>"
  Bus Selector/5 -> Compare To Constant4/1  "<MCU2_5ldcSensorFault>"
  Bus Selector/4 -> Compare To Constant3/1  "<MCU2_5ActiveDischargingFault>"
  Bus Selector/3 -> Compare To Constant2/1  "<MCU2_5TempSensorFault>"
  Bus Selector/2 -> Compare To Constant1/1  "<MCU2_5UdcDetectionFault>"
  Bus Selector/1 -> Compare To Constant/1  "<MCU2_5MotorStallingFault>"
  MCU2_5/1 -> Bus Selector/1

== system six_plus_six_AcmsteeringV09_main_2lflm/MainControl/mode_control/forward/forward/Brake/Switch Case Action Subsystem ==
  bratrq_dem_lf : Inport
  bratrq_dem_lm : Inport  Port=2
  bratrq_dem_lr : Inport  Port=3
  bratrq_dem_rf : Inport  Port=4
  bratrq_dem_rm : Inport  Port=5
  bratrq_dem_rr : Inport  Port=6
  pwr_chg_bat : Inport  Port=7
  pwr_chg_bat1 : Inport  Port=8
  pwr_chg_bat2 : Inport  Port=9
  trqlimL_dig_lf : Inport  Port=10
  trqlimL_dig_lm : Inport  Port=11
  trqlimL_dig_lr : Inport  Port=12
  trqlimL_dig_rf : Inport  Port=13
  trqlimL_dig_rm : Inport  Port=14
  trqlimL_dig_rr : Inport  Port=15
  speed_act_lf : Inport  Port=16
  speed_act_lm : Inport  Port=17
  speed_act_lr : Inport  Port=18
  speed_act_rf : Inport  Port=19
  speed_act_rm : Inport  Port=20
  speed_act_rr : Inport  Port=21
  trqlim_map_lf : Inport  Port=22
  trqlim_map_lm : Inport  Port=23
  trqlim_map_lr : Inport  Port=24
  trqlim_map_rf : Inport  Port=25
  trqlim_map_rm : Inport  Port=26
  trqlim_map_rr : Inport  Port=27
  tras_ratio : Inport  Port=28
  guzhang_lf : Inport  Port=29
  guzhang_lm : Inport  Port=30
  guzhang_lr : Inport  Port=31
  guzhang_rf : Inport  Port=32
  guzhang_rm : Inport  Port=33
  guzhang_rr : Inport  Port=34
  MATLAB Function5 : MATLAB Function  TreatAsAtomicUnit=on
  bratrq_mot_lf : Outport
  bratrq_mot_lm : Outport  Port=2
  bratrq_mot_lr : Outport  Port=3
  bratrq_mot_rf : Outport  Port=4
  bratrq_mot_rm : Outport  Port=5
  bratrq_mot_rr : Outport  Port=6
  brapre_out_l : Outport  Port=7
  brapre_out_r : Outport  Port=8
  wires:
  MATLAB Function5/3(bratrq_mot_lr) -> bratrq_mot_lr/1
  MATLAB Function5/1(bratrq_mot_lf) -> bratrq_mot_lf/1
  MATLAB Function5/2(bratrq_mot_lm) -> bratrq_mot_lm/1
  MATLAB Function5/8(brapre_out_r) -> brapre_out_r/1
  MATLAB Function5/4(bratrq_mot_rf) -> bratrq_mot_rf/1
  MATLAB Function5/7(brapre_out_l) -> brapre_out_l/1
  MATLAB Function5/6(bratrq_mot_rr) -> bratrq_mot_rr/1
  MATLAB Function5/5(bratrq_mot_rm) -> bratrq_mot_rm/1
  bratrq_dem_lf/1 -> MATLAB Function5/1(bratrq_dem_lf)
  bratrq_dem_lm/1 -> MATLAB Function5/2(bratrq_dem_lm)
  bratrq_dem_lr/1 -> MATLAB Function5/3(bratrq_dem_lr)
  bratrq_dem_rf/1 -> MATLAB Function5/4(bratrq_dem_rf)
  bratrq_dem_rm/1 -> MATLAB Function5/5(bratrq_dem_rm)
  bratrq_dem_rr/1 -> MATLAB Function5/6(bratrq_dem_rr)
  pwr_chg_bat/1 -> MATLAB Function5/7(pwr_chg_bat)
  pwr_chg_bat1/1 -> MATLAB Function5/8(pwr_chg_bat1)
  pwr_chg_bat2/1 -> MATLAB Function5/9(pwr_chg_bat2)
  trqlimL_dig_lf/1 -> MATLAB Function5/10(trqlimL_dig_lf)
  trqlimL_dig_lm/1 -> MATLAB Function5/11(trqlimL_dig_lm)
  trqlimL_dig_lr/1 -> MATLAB Function5/12(trqlimL_dig_lr)
  trqlimL_dig_rf/1 -> MATLAB Function5/13(trqlimL_dig_rf)
  trqlimL_dig_rm/1 -> MATLAB Function5/14(trqlimL_dig_rm)
  speed_act_lf/1 -> MATLAB Function5/16(speed_act_lf)
  trqlimL_dig_rr/1 -> MATLAB Function5/15(trqlimL_dig_rr)
  speed_act_lm/1 -> MATLAB Function5/17(speed_act_lm)
  speed_act_lr/1 -> MATLAB Function5/18(speed_act_lr)
  speed_act_rf/1 -> MATLAB Function5/19(speed_act_rf)
  speed_act_rm/1 -> MATLAB Function5/20(speed_act_rm)
  speed_act_rr/1 -> MATLAB Function5/21(speed_act_rr)
  trqlim_map_lm/1 -> MATLAB Function5/23(trqlim_map_lm)
  trqlim_map_lf/1 -> MATLAB Function5/22(trqlim_map_lf)
  trqlim_map_lr/1 -> MATLAB Function5/24(trqlim_map_lr)
  trqlim_map_rf/1 -> MATLAB Function5/25(trqlim_map_rf)
  trqlim_map_rm/1 -> MATLAB Function5/26(trqlim_map_rm)
  trqlim_map_rr/1 -> MATLAB Function5/27(trqlim_map_rr)
  tras_ratio/1 -> MATLAB Function5/28(tras_ratio)
  guzhang_lf/1 -> MATLAB Function5/29(guzhang_lf)
  guzhang_lm/1 -> MATLAB Function5/30(guzhang_lm)
  guzhang_lr/1 -> MATLAB Function5/31(guzhang_lr)
  guzhang_rf/1 -> MATLAB Function5/32(guzhang_rf)
  guzhang_rm/1 -> MATLAB Function5/33(guzhang_rm)
  guzhang_rr/1 -> MATLAB Function5/34(guzhang_rr)

== system six_plus_six_AcmsteeringV09_main_2lflm/MainControl/mode_control/forward/forward/Drive/Subsystem ==
  MCU2 : Inport
  Bus Selector : BusSelector  OutputSignals=MCU2_MotorStallingFault,MCU2_UdcDetectionFault,MCU2_TempSensorFault,MCU2_ActiveDischargingFault,MCU2_ldcSensorFault,MCU2_luSensorFault,MCU2_lvSensorFault,MCU2_FaultLevel,MCU2_Controllerload,MCU2_CanCommunicationFault,MCU2_MemoryFault,MCU2_DownratingFault,MCU2_IGBTFault,MCU2_MotorOverTemp,MCU2_ControllerOverTemp,MCU2_MotorOverSpeed,MCU2_RotaryInverterFault,MCU2_UnderVoltage,MCU2_OverVoltage,MCU2_MotorOverLoad
  Compare To Constant{,1..19} (20 alike) : simulink/Logic and Bit Operations/Compare To Constant  relop===  const=1  OutDataTypeStr=boolean
  Logical Operator : Logic  Operator=OR  Inputs=20  AllPortsSameDT=off  OutDataTypeStr=boolean
  guzhang_lf : Outport
  wires:
  MCU2/1 -> Bus Selector/1
  Bus Selector/1 -> Compare To Constant/1  "<MCU2_MotorStallingFault>"
  Bus Selector/2 -> Compare To Constant1/1  "<MCU2_UdcDetectionFault>"
  Bus Selector/3 -> Compare To Constant2/1  "<MCU2_TempSensorFault>"
  Bus Selector/4 -> Compare To Constant3/1  "<MCU2_ActiveDischargingFault>"
  Bus Selector/5 -> Compare To Constant4/1  "<MCU2_ldcSensorFault>"
  Bus Selector/6 -> Compare To Constant5/1  "<MCU2_luSensorFault>"
  Bus Selector/7 -> Compare To Constant6/1  "<MCU2_lvSensorFault>"
  Bus Selector/8 -> Compare To Constant7/1  "<MCU2_FaultLevel>"
  Bus Selector/13 -> Compare To Constant12/1  "<MCU2_IGBTFault>"
  Bus Selector/14 -> Compare To Constant13/1  "<MCU2_MotorOverTemp>"
  Bus Selector/10 -> Compare To Constant9/1  "<MCU2_CanCommunicationFault>"
  Bus Selector/16 -> Compare To Constant15/1  "<MCU2_MotorOverSpeed>"
  Bus Selector/11 -> Compare To Constant10/1  "<MCU2_MemoryFault>"
  Bus Selector/15 -> Compare To Constant14/1  "<MCU2_ControllerOverTemp>"
  Bus Selector/12 -> Compare To Constant11/1  "<MCU2_DownratingFault>"
  Bus Selector/9 -> Compare To Constant8/1  "<MCU2_Controllerload>"
  Bus Selector/18 -> Compare To Constant17/1  "<MCU2_UnderVoltage>"
  Bus Selector/20 -> Compare To Constant19/1  "<MCU2_MotorOverLoad>"
  Bus Selector/19 -> Compare To Constant18/1  "<MCU2_OverVoltage>"
  Bus Selector/17 -> Compare To Constant16/1  "<MCU2_RotaryInverterFault>"
  Compare To Constant9/1 -> Logical Operator/10
  Compare To Constant12/1 -> Logical Operator/13
  Compare To Constant11/1 -> Logical Operator/12
  Compare To Constant15/1 -> Logical Operator/16
  Compare To Constant8/1 -> Logical Operator/9
  Compare To Constant10/1 -> Logical Operator/11
  Compare To Constant13/1 -> Logical Operator/14
  Compare To Constant14/1 -> Logical Operator/15
  Compare To Constant1/1 -> Logical Operator/2
  Compare To Constant17/1 -> Logical Operator/18
  Compare To Constant16/1 -> Logical Operator/17
  Compare To Constant18/1 -> Logical Operator/19
  Compare To Constant19/1 -> Logical Operator/20
  Compare To Constant3/1 -> Logical Operator/4
  Compare To Constant2/1 -> Logical Operator/3
  Compare To Constant6/1 -> Logical Operator/7
  Compare To Constant4/1 -> Logical Operator/5
  Compare To Constant5/1 -> Logical Operator/6
  Compare To Constant7/1 -> Logical Operator/8
  Compare To Constant/1 -> Logical Operator/1
  Logical Operator/1 -> guzhang_lf/1

== system six_plus_six_AcmsteeringV09_main_2lflm/MainControl/mode_control/forward/forward/Drive/Subsystem1 ==
  MCU2_2 : Inport
  Bus Selector : BusSelector  OutputSignals=MCU2_2MotorStallingFault,MCU2_2UdcDetectionFault,MCU2_2TempSensorFault,MCU2_2ActiveDischargingFault,MCU2_2ldcSensorFault,MCU2_2luSensorFault,MCU2_2lvSensorFault,MCU2_2FaultLevel,MCU2_2Controllerload,MCU2_2CanCommunicationFault,MCU2_2MemoryFault,MCU2_2DownratingFault,MCU2_2IGBTFault,MCU2_2MotorOverTemp,MCU2_2ControllerOverTemp,MCU2_2MotorOverSpeed,MCU2_2RotaryInverterFault,MCU2_2UnderVoltage,MCU2_OverVoltage,MCU2_2MotorOverLoad
  Compare To Constant{,1..19} (20 alike) : simulink/Logic and Bit Operations/Compare To Constant  relop===  const=1  OutDataTypeStr=boolean
  Logical Operator : Logic  Operator=OR  Inputs=20  AllPortsSameDT=off  OutDataTypeStr=boolean
  guzhang_lm : Outport
  wires:
  Logical Operator/1 -> guzhang_lm/1
  Compare To Constant/1 -> Logical Operator/1
  Compare To Constant7/1 -> Logical Operator/8
  Compare To Constant5/1 -> Logical Operator/6
  Compare To Constant4/1 -> Logical Operator/5
  Compare To Constant6/1 -> Logical Operator/7
  Compare To Constant2/1 -> Logical Operator/3
  Compare To Constant3/1 -> Logical Operator/4
  Compare To Constant19/1 -> Logical Operator/20
  Compare To Constant18/1 -> Logical Operator/19
  Compare To Constant16/1 -> Logical Operator/17
  Compare To Constant17/1 -> Logical Operator/18
  Compare To Constant1/1 -> Logical Operator/2
  Compare To Constant14/1 -> Logical Operator/15
  Compare To Constant13/1 -> Logical Operator/14
  Compare To Constant10/1 -> Logical Operator/11
  Compare To Constant8/1 -> Logical Operator/9
  Compare To Constant15/1 -> Logical Operator/16
  Compare To Constant11/1 -> Logical Operator/12
  Compare To Constant12/1 -> Logical Operator/13
  Compare To Constant9/1 -> Logical Operator/10
  Bus Selector/17 -> Compare To Constant16/1  "<MCU2_2RotaryInverterFault>"
  Bus Selector/19 -> Compare To Constant18/1  "<MCU2_OverVoltage>"
  Bus Selector/20 -> Compare To Constant19/1  "<MCU2_2MotorOverLoad>"
  Bus Selector/18 -> Compare To Constant17/1  "<MCU2_2UnderVoltage>"
  Bus Selector/9 -> Compare To Constant8/1  "<MCU2_2Controllerload>"
  Bus Selector/12 -> Compare To Constant11/1  "<MCU2_2DownratingFault>"
  Bus Selector/15 -> Compare To Constant14/1  "<MCU2_2ControllerOverTemp>"
  Bus Selector/11 -> Compare To Constant10/1  "<MCU2_2MemoryFault>"
  Bus Selector/16 -> Compare To Constant15/1  "<MCU2_2MotorOverSpeed>"
  Bus Selector/10 -> Compare To Constant9/1  "<MCU2_2CanCommunicationFault>"
  Bus Selector/14 -> Compare To Constant13/1  "<MCU2_2MotorOverTemp>"
  Bus Selector/13 -> Compare To Constant12/1  "<MCU2_2IGBTFault>"
  Bus Selector/8 -> Compare To Constant7/1  "<MCU2_2FaultLevel>"
  Bus Selector/7 -> Compare To Constant6/1  "<MCU2_2lvSensorFault>"
  Bus Selector/6 -> Compare To Constant5/1  "<MCU2_2luSensorFault>"
  Bus Selector/5 -> Compare To Constant4/1  "<MCU2_2ldcSensorFault>"
  Bus Selector/4 -> Compare To Constant3/1  "<MCU2_2ActiveDischargingFault>"
  Bus Selector/3 -> Compare To Constant2/1  "<MCU2_2TempSensorFault>"
  Bus Selector/2 -> Compare To Constant1/1  "<MCU2_2UdcDetectionFault>"
  Bus Selector/1 -> Compare To Constant/1  "<MCU2_2MotorStallingFault>"
  MCU2_2/1 -> Bus Selector/1
